simulink model "lqr_final"  (R2018a)
settings: Solver=VariableStepAuto  StartTime=0.0  StopTime=500  RelTol=1e-3
values from neighbouring files (symbols this model uses):
  D = 0    [k_func.m]
libraries: simulink_extras x5, sharedutil x2, dspmtrx3 x1
settings Model: Creator=Renz  LastModifiedBy=Renz

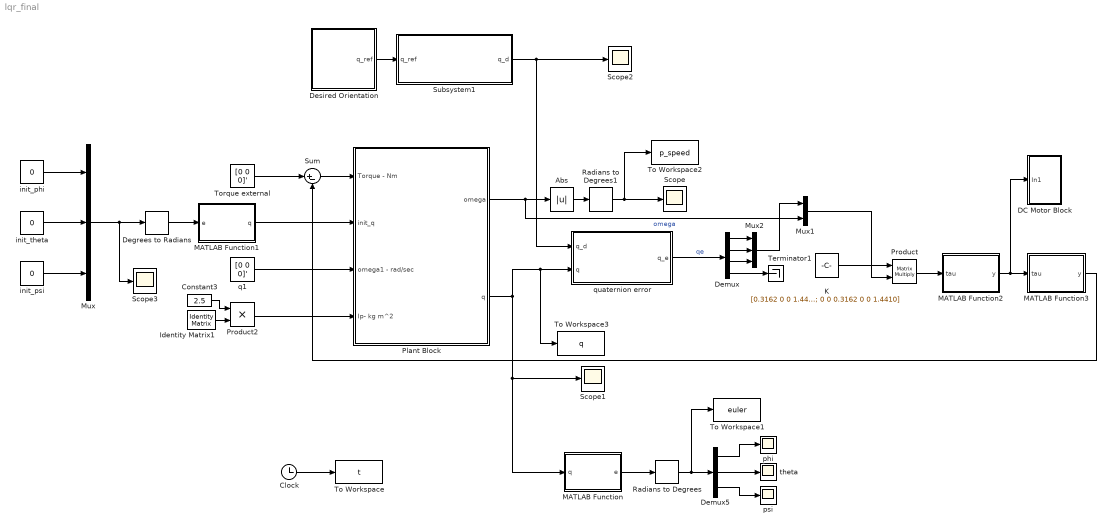
== system lqr_final ==
  Abs : Abs
  Clock : Clock
  Constant3 : Constant  Value=2.5
  DC Motor Block : Subsystem
  Degrees to Radians : simulink_extras/Transformations/Degrees to Radians
  Demux : Demux
  Demux5 : Demux  Outputs=3
  Desired Orientation : Subsystem
  Identity Matrix1 : dspmtrx3/Identity Matrix  Inherit=off  N=3  Ts=1  dataType=double  isSigned=on  wordLen=16  udDataType=sfix(16)  fracBitsMode=Best precision  numFracBits=15  OutDataTypeStr=double  LastOutDataTypeStr=double
      settings: SourceProductName=DSP System Toolbox
  K : Constant  Value=[0.3162 0 0 1.4410 0 0; 0 0.3162 0 0 1.4410 0; 0 0 0.3162 0 0 1.4410]
  MATLAB Function : MATLAB Function  TreatAsAtomicUnit=on
  MATLAB Function1 : MATLAB Function  TreatAsAtomicUnit=on
  MATLAB Function2 : MATLAB Function  TreatAsAtomicUnit=on
  MATLAB Function3 : MATLAB Function  TreatAsAtomicUnit=on
  Mux : Mux  Inputs=3
  Mux1 : Mux  Inputs=2
  Mux2 : Mux  Inputs=3
  Plant Block : Subsystem
  Product : Product  Multiplication=Matrix(*)
  Product2 : Product
  Radians to Degrees : simulink_extras/Transformations/Radians to Degrees
  Radians to Degrees1 : simulink_extras/Transformations/Radians to Degrees
  Scope{,1..3} (4 alike) : Scope
  Subsystem1 : Subsystem
  Sum : Sum  Inputs=|+-
  Terminator1 : Terminator
  To Workspace : ToWorkspace  VariableName=t  SampleTime=-1
  To Workspace1 : ToWorkspace  VariableName=euler  SampleTime=-1
  To Workspace2 : ToWorkspace  VariableName=p_speed  SampleTime=-1
  To Workspace3 : ToWorkspace  VariableName=q  SampleTime=-1
  Torque external : Constant  Value=[0 0 0]'
  init_phi : Constant  Value=0
  init_psi : Constant  Value=0
  init_theta : Constant  Value=0
  phi : Scope
  psi : Scope
  q1 : Constant  Value=[0 0 0]'
  quaternion error : Subsystem
  theta : Scope
  wires:
  MATLAB Function/1(e) -> Radians to Degrees/1
  Degrees to Radians/1 -> MATLAB Function1/1(e)
  Demux5/2 -> theta/1
  init_psi/1 -> Mux/3
  Plant Block/2(q) -> To Workspace3/1, quaternion error/2(q), MATLAB Function/1(q), Scope1/1
  Subsystem1/1(q_d) -> quaternion error/1(q_d), Scope2/1
  Demux5/1 -> phi/1
  Sum/1 -> Plant Block/1(Torque - Nm)
  Desired Orientation/1(q_ref) -> Subsystem1/1(q_ref)
  Constant3/1 -> Product2/1
  MATLAB Function1/1(q) -> Plant Block/2(init_q)
  Torque external/1 -> Sum/1
  Clock/1 -> To Workspace/1
  init_theta/1 -> Mux/2
  quaternion error/1(q_e) -> Demux/1  "qe"
  q1/1 -> Plant Block/3(omega1 - rad/sec)
  Plant Block/1(omega) -> Abs/1, Mux1/2  "omega"
  Radians to Degrees/1 -> To Workspace1/1, Demux5/1
  Mux/1 -> Scope3/1, Degrees to Radians/1
  Product2/1 -> Plant Block/4(Ip- kg m^2)
  Identity Matrix1/1 -> Product2/2
  Demux5/3 -> psi/1
  MATLAB Function2/1(y) -> DC Motor Block/1(In1), MATLAB Function3/1(tau)
  init_phi/1 -> Mux/1
  Mux1/1 -> Product/2
  Abs/1 -> Radians to Degrees1/1
  Product/1 -> MATLAB Function2/1(tau)
  MATLAB Function3/1(y) -> Sum/2
  Demux/2 -> Mux2/2
  Demux/1 -> Mux2/1
  Demux/3 -> Mux2/3
  Mux2/1 -> Mux1/1
  K/1 -> Product/1
  Demux/4 -> Terminator1/1
  Radians to Degrees1/1 -> Scope/1, To Workspace2/1

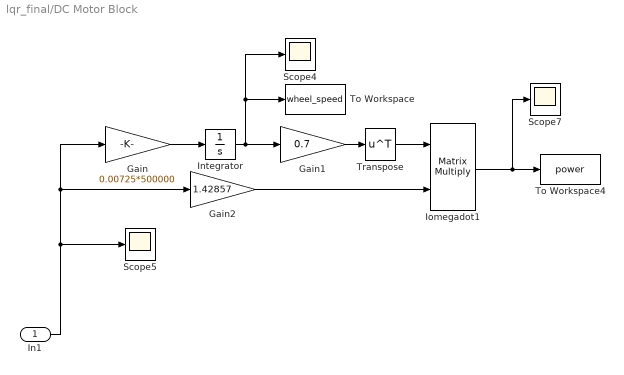
== system lqr_final/DC Motor Block ==
  In1 : Inport
  Gain : Gain  Gain=0.00725*500000
  Gain1 : Gain  Gain=0.7
  Gain2 : Gain  Gain=1.42857
  Integrator : Integrator
  Iomegadot1 : Product  Multiplication=Matrix(*)
  Scope4 : Scope
  Scope5 : Scope
  Scope7 : Scope
  To Workspace : ToWorkspace  VariableName=wheel_speed  SampleTime=-1
  To Workspace4 : ToWorkspace  VariableName=power  SampleTime=-1
  Transpose : Math  Operator=transpose  SaturateOnIntegerOverflow=on
  wires:
  Gain/1 -> Integrator/1
  Gain2/1 -> Iomegadot1/2
  Iomegadot1/1 -> Scope7/1, To Workspace4/1
  Transpose/1 -> Iomegadot1/1
  In1/1 -> Scope5/1, Gain2/1, Gain/1
  Integrator/1 -> To Workspace/1, Scope4/1, Gain1/1
  Gain1/1 -> Transpose/1

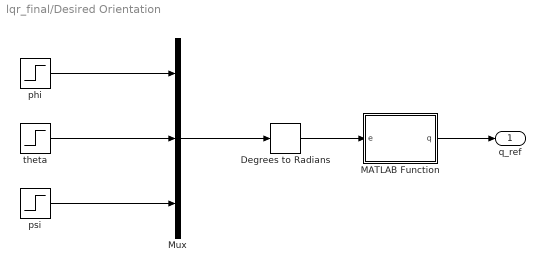
== system lqr_final/Desired Orientation ==
  Degrees to Radians : simulink_extras/Transformations/Degrees to Radians
  MATLAB Function : MATLAB Function  TreatAsAtomicUnit=on
  Mux : Mux  Inputs=3
  phi : Step  After=10  SampleTime=0
  psi : Step  After=30  SampleTime=0
  theta : Step  After=15  SampleTime=0
  q_ref : Outport
  wires:
  Mux/1 -> Degrees to Radians/1
  psi/1 -> Mux/3
  phi/1 -> Mux/1
  theta/1 -> Mux/2
  MATLAB Function/1(q) -> q_ref/1
  Degrees to Radians/1 -> MATLAB Function/1(e)

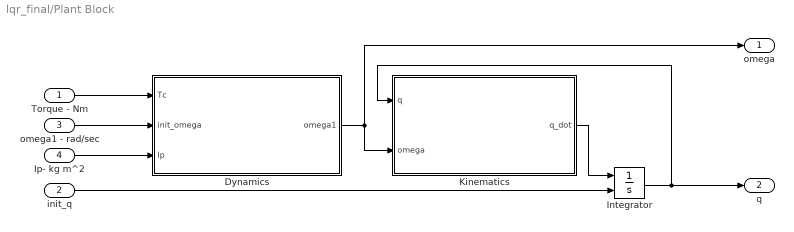
== system lqr_final/Plant Block ==
  Torque - Nm : Inport
  init_q : Inport  Port=2
  omega1 - rad/sec : Inport  Port=3
  Ip- kg m^2 : Inport  Port=4
  Dynamics : Subsystem
  Integrator : Integrator  InitialConditionSource=external
  Kinematics : Subsystem
  omega : Outport
  q : Outport  Port=2
  wires:
  Kinematics/1(q_dot) -> Integrator/1
  Integrator/1 -> Kinematics/1(q), q/1
  Torque - Nm/1 -> Dynamics/1(Tc)
  omega1 - rad/sec/1 -> Dynamics/2(init_omega)
  init_q/1 -> Integrator/2
  Dynamics/1(omega1) -> Kinematics/2(omega), omega/1
  Ip- kg m^2/1 -> Dynamics/3(Ip)

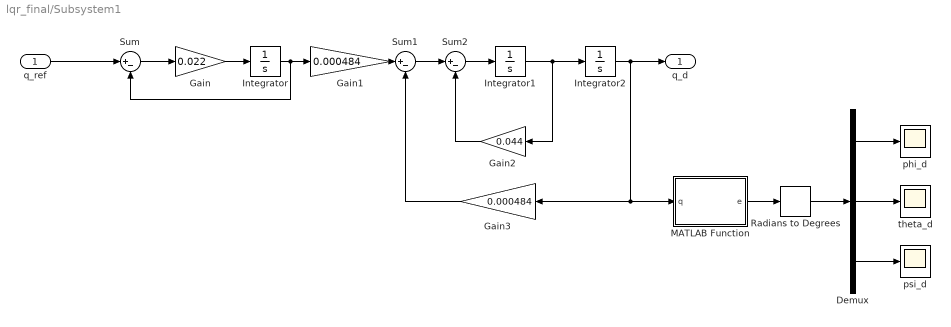
== system lqr_final/Subsystem1 ==
  q_ref : Inport
  Demux : Demux  Outputs=3
  Gain : Gain  Gain=0.022
  Gain1 : Gain  Gain=0.000484
  Gain2 : Gain  Gain=0.044
  Gain3 : Gain  Gain=0.000484
  Integrator : Integrator
  Integrator1 : Integrator
  Integrator2 : Integrator
  MATLAB Function : MATLAB Function  TreatAsAtomicUnit=on
  Radians to Degrees : simulink_extras/Transformations/Radians to Degrees
  Sum : Sum  Inputs=|+-
  Sum1 : Sum  Inputs=|+-
  Sum2 : Sum  Inputs=|+-
  phi_d : Scope
  psi_d : Scope
  theta_d : Scope
  q_d : Outport
  wires:
  Demux/3 -> psi_d/1
  Gain1/1 -> Sum1/1
  Sum/1 -> Gain/1
  Gain2/1 -> Sum2/2
  Demux/2 -> theta_d/1
  Gain/1 -> Integrator/1
  Integrator/1 -> Gain1/1, Sum/2
  Sum1/1 -> Sum2/1
  Gain3/1 -> Sum1/2
  Integrator1/1 -> Gain2/1, Integrator2/1
  Sum2/1 -> Integrator1/1
  q_ref/1 -> Sum/1
  Demux/1 -> phi_d/1
  Radians to Degrees/1 -> Demux/1
  Integrator2/1 -> q_d/1, MATLAB Function/1(q), Gain3/1
  MATLAB Function/1(e) -> Radians to Degrees/1

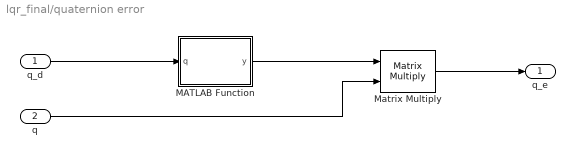
== system lqr_final/quaternion error ==
  q_d : Inport
  q : Inport  Port=2
  MATLAB Function : MATLAB Function  TreatAsAtomicUnit=on
  Matrix Multiply : Product  Multiplication=Matrix(*)
  q_e : Outport
  wires:
  MATLAB Function/1(y) -> Matrix Multiply/1
  Matrix Multiply/1 -> q_e/1
  q/1 -> Matrix Multiply/2
  q_d/1 -> MATLAB Function/1(q)

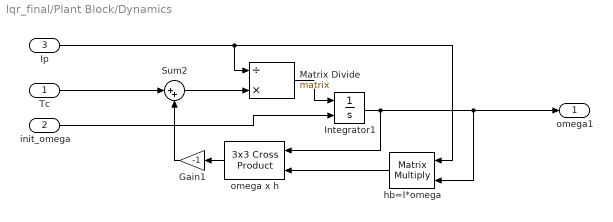
== system lqr_final/Plant Block/Dynamics ==
  Tc : Inport
  init_omega : Inport  Port=2
  Ip : Inport  Port=3
  Gain1 : Gain  Gain=-1
  Integrator1 : Integrator  InitialConditionSource=external  ZeroCross=off
  Matrix Divide : Product  Inputs=/*  Multiplication=Matrix(*)
  Sum2 : Sum  Inputs=|++
  hb=I*omega : Product  Multiplication=Matrix(*)
  omega x h : sharedutil/3x3 Cross Product  aMode=aMode
      settings: SourceProductBaseCode=AE
  omega1 : Outport
  wires:
  Gain1/1 -> Sum2/2
  Integrator1/1 -> omega x h/1, omega1/1, hb=I*omega/2
  init_omega/1 -> Integrator1/2
  Sum2/1 -> Matrix Divide/2
  hb=I*omega/1 -> omega x h/2
  omega x h/1 -> Gain1/1
  Tc/1 -> Sum2/1
  Matrix Divide/1 -> Integrator1/1
  Ip/1 -> Matrix Divide/1, hb=I*omega/1

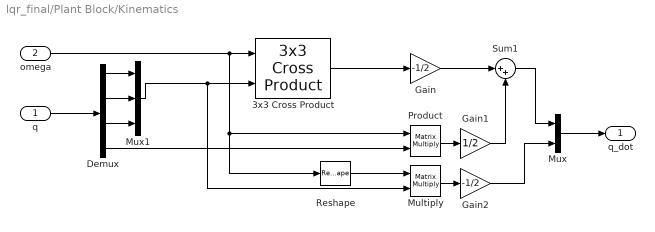
== system lqr_final/Plant Block/Kinematics ==
  q : Inport
  omega : Inport  Port=2
  3x3 Cross Product : sharedutil/3x3 Cross Product  aMode=aMode
      settings: SourceProductBaseCode=AE
  Demux : Demux
  Gain : Gain  Gain=-1/2
  Gain1 : Gain  Gain=1/2
  Gain2 : Gain  Gain=-1/2
  Multiply : Product  Multiplication=Matrix(*)
  Mux : Mux  Inputs=2
  Mux1 : Mux  Inputs=3
  Product : Product  Multiplication=Matrix(*)
  Reshape : Reshape  OutputDimensionality=Row vector (2-D)
  Sum1 : Sum  Inputs=|++
  q_dot : Outport
  wires:
  omega/1 -> 3x3 Cross Product/1, Product/1, Reshape/1
  Mux1/1 -> Multiply/2, 3x3 Cross Product/2
  Gain1/1 -> Sum1/2
  3x3 Cross Product/1 -> Gain/1
  Product/1 -> Gain1/1
  Multiply/1 -> Gain2/1
  Gain/1 -> Sum1/1
  Demux/4 -> Product/2
  Sum1/1 -> Mux/1
  Gain2/1 -> Mux/2
  Reshape/1 -> Multiply/1
  Mux/1 -> q_dot/1
  Demux/1 -> Mux1/1
  q/1 -> Demux/1
  Demux/2 -> Mux1/2
  Demux/3 -> Mux1/3

== matlab function lqr_final/Subsystem1/MATLAB Function ==
  data: q input; e output
function e = quat2euler(q)

q0 = q(1,:);
q1 = q(2,:);
q2 = q(3,:);
q3 = q(4,:);

phi = atan((2*(q2*q3 + q0*q1))/(q0^2 - q1^2 - q2^2 + q3^2)); 
theta = asin(-2*(q1*q3 - q0*q2));
psi = atan((2*(q1*q2 + q0*q3))/(q0^2 + q1^2 -q2^2 - q3^2)); 

e = [phi;theta;psi];

end

== matlab function lqr_final/Desired Orientation/MATLAB Function ==
  data: e input; q output
function q = euler2quat(e)

e1 = 0.5*e(1,:);
e2 = 0.5*e(2,:);
e3 = 0.5*e(3,:);

q0 = (sin(e1)*sin(e2)*sin(e3)) + (cos(e1)*cos(e2)*cos(e3));
q1 = (-sin(e2)*sin(e3)*cos(e1)) + (sin(e1)*cos(e2)*cos(e3));
q2 = (sin(e1)*cos(e2)*sin(e3)) + (sin(e2)*cos(e1)*cos(e3));
q3 = (sin(e3)*cos(e1)*cos(e2)) - (sin(e1)*sin(e2)*cos(e3));

q = [q0;q1;q2;q3];

end

== matlab function lqr_final/MATLAB Function1 ==
  data: e input; q output
function q = euler2quat(e)

e1 = 0.5*e(1,:);
e2 = 0.5*e(2,:);
e3 = 0.5*e(3,:);

q0 = (sin(e1)*sin(e2)*sin(e3)) + (cos(e1)*cos(e2)*cos(e3));
q1 = (-sin(e2)*sin(e3)*cos(e1)) + (sin(e1)*cos(e2)*cos(e3));
q2 = (sin(e1)*cos(e2)*sin(e3)) + (sin(e2)*cos(e1)*cos(e3));
q3 = (sin(e3)*cos(e1)*cos(e2)) - (sin(e1)*sin(e2)*cos(e3));

q = [q0;q1;q2;q3];

end

== matlab function lqr_final/MATLAB Function3 ==
  data: tau input; y output
function y = torque(tau)
L = [0.57735, -0.57735, -0.57735, 0.57735; 0.57735, -0.57735, 0.57735, -0.57735; 0.57735, 0.57735, -0.57735, -0.57735];


y = L*tau;

== matlab function lqr_final/quaternion error/MATLAB Function ==
  data: q input; y output
function y = q_error(q)
q1 = q(1,:);
q2 = q(2,:);
q3 = q(3,:);
q4 = q(4,:);

y = [q4,q3,-q2,-q1; -q3,q4,q1,-q2; q2,-q1,q4,-q3; q1,q2,q3,q4];

== matlab function lqr_final/MATLAB Function ==
  data: q input; e output
function e = quat2euler(q)

q0 = q(1,:);
q1 = q(2,:);
q2 = q(3,:);
q3 = q(4,:);

phi = atan((2*(q2*q3 + q0*q1))/(q0^2 - q1^2 - q2^2 + q3^2)); 
theta = asin(-2*(q1*q3 - q0*q2));
psi = atan((2*(q1*q2 + q0*q3))/(q0^2 + q1^2 -q2^2 - q3^2)); 

e = [phi;theta;psi];

end

== matlab function lqr_final/MATLAB Function2 ==
  data: tau input; y output
function y = control_alloc(tau)
K =[1 0 0 0 
    0 1 0 0 
    0 0 1 0 
    0 0 0 1];
T = [0.57735, -0.57735, -0.57735, 0.57735; 0.57735, -0.57735, 0.57735, -0.57735; 0.57735, 0.57735, -0.57735, -0.57735];
W = [1 0 0 0     
    0 1 0 0      
    0 0 1 0      
    0 0 0 1];


y = ucalloc(K,T,W,tau);
